simulink model "test_coremath"  (R2020b)
settings: Solver=VariableStepAuto  StartTime=0.0  StopTime=10.0  RelTol=1e-3
undefined symbols (not defined in the file): mergepose
libraries: simlib_vpc_coremath x12, dspinverses x1
settings Model: Creator=marco  LastModifiedBy=marco

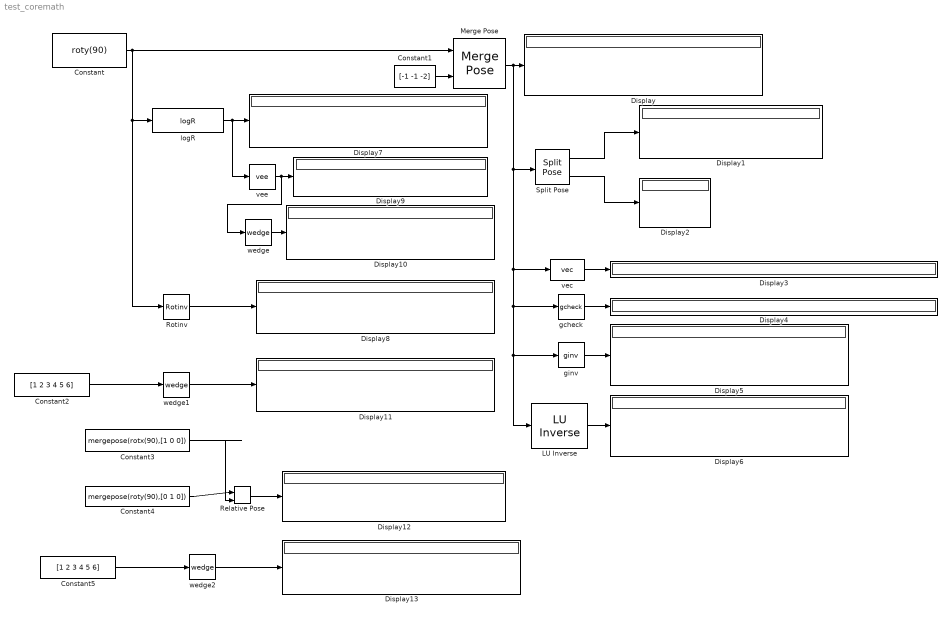
== system test_coremath ==
  " LU Inverse" : dspinverses/ LU Inverse
  Constant : Constant  Value=roty(90)
  Constant1 : Constant  Value=[-1 -1 -2]
  Constant2 : Constant  Value=[1 2 3 4 5 6]
  Constant3 : Constant  Value=mergepose(rotx(90),[1 0 0])
  Constant4 : Constant  Value=mergepose(roty(90),[0 1 0])
  Constant5 : Constant  Value=[1 2 3 4 5 6]
  Display{,1..13} (14 alike) : Display
  Merge Pose : simlib_vpc_coremath/Merge Pose
      settings: SourceProductName=VPC Library
  Relative Pose : simlib_vpc_coremath/Relative Pose
      settings: SourceProductName=VPC Library
  Rotinv : simlib_vpc_coremath/Rotinv
      settings: SourceProductName=VPC Library
  Split Pose : simlib_vpc_coremath/Split Pose
      settings: SourceProductName=VPC Library
  gcheck : simlib_vpc_coremath/gcheck
      settings: SourceProductName=VPC Library
  ginv : simlib_vpc_coremath/ginv
      settings: SourceProductName=VPC Library
  logR : simlib_vpc_coremath/logR
      settings: SourceProductName=VPC Library
  vec : simlib_vpc_coremath/vec
      settings: SourceProductName=VPC Library
  vee : simlib_vpc_coremath/vee
      settings: SourceProductName=VPC Library
  wedge : simlib_vpc_coremath/wedge
      settings: SourceProductName=VPC Library
  wedge1 : simlib_vpc_coremath/wedge
      settings: SourceProductName=VPC Library
  wedge2 : simlib_vpc_coremath/wedge
      settings: SourceProductName=VPC Library
  wires:
  Merge Pose/1 -> " LU Inverse"/1, ginv/1, gcheck/1, vec/1, Split Pose/1, Display/1
  Constant/1 -> Rotinv/1, logR/1, Merge Pose/1
  Constant1/1 -> Merge Pose/2
  Split Pose/1 -> Display1/1
  Split Pose/2 -> Display2/1
  vec/1 -> Display3/1
  gcheck/1 -> Display4/1
  ginv/1 -> Display5/1
  " LU Inverse"/1 -> Display6/1
  logR/1 -> vee/1, Display7/1
  Rotinv/1 -> Display8/1
  vee/1 -> wedge/1, Display9/1
  wedge/1 -> Display10/1
  Constant2/1 -> wedge1/1
  wedge1/1 -> Display11/1
  Constant4/1 -> Relative Pose/1
  Constant3/1 -> Relative Pose/2
  Relative Pose/1 -> Display12/1
  Constant5/1 -> wedge2/1
  wedge2/1 -> Display13/1
